simulink model "TRLQR2"  (R2024b)
settings: Solver=VariableStepAuto  StartTime=0.0  StopTime=10.0  RelTol=1e-3
undefined symbols (not defined in the file): start, theta0
settings Model: Creator=mwali  LastModifiedBy=mwali
settings ConfigComp: CovBoundaryAbsTol=1.0e-5

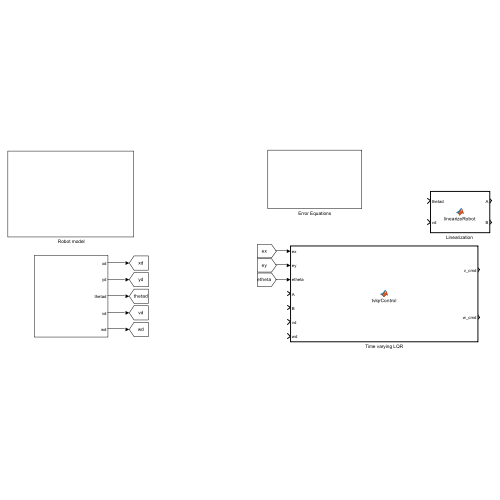
[thumbnail: Simulink's stored preview of the top-level diagram]
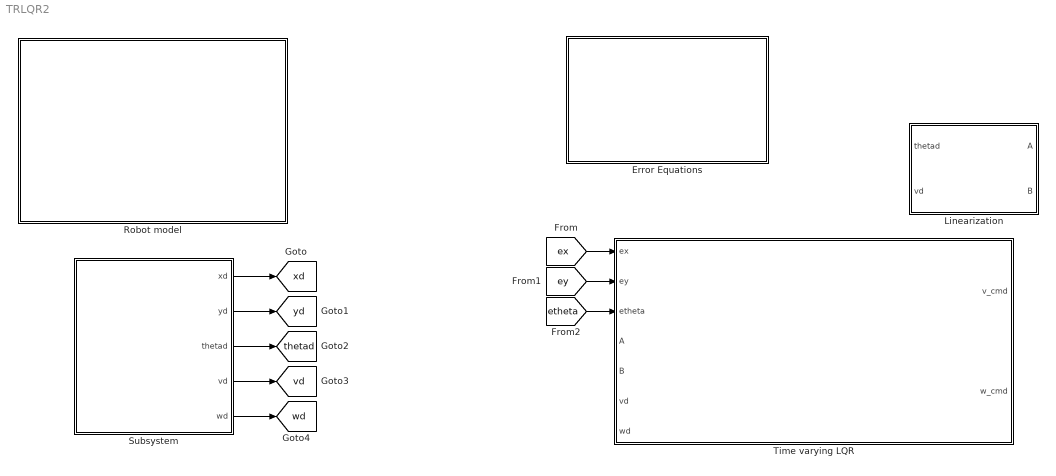
== system TRLQR2 ==
  " Robot model" : Subsystem
  Error Equations : Subsystem
  "Linearization " : MATLAB Function  TreatAsAtomicUnit=on
  Subsystem : Subsystem
  Time varying LQR : MATLAB Function  TreatAsAtomicUnit=on
  tag scope: thetad=global, vd=global, wd=global, xd=global, yd=global
  wires:
  [ex] -> Time varying LQR/1(ex)
  [ey] -> Time varying LQR/2(ey)
  [etheta] -> Time varying LQR/3(etheta)
  Subsystem/1(xd) -> [xd]
  Subsystem/2(yd) -> [yd]
  Subsystem/3(thetad) -> [thetad]
  Subsystem/4(vd) -> [vd]
  Subsystem/5(wd) -> [wd]

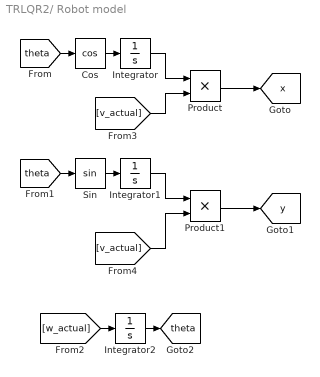
== system TRLQR2/ Robot model ==
  Cos : Trigonometry  Operator=cos
  Integrator : Integrator  InitialCondition=start(1)
  Integrator1 : Integrator  InitialCondition=start(2)
  Integrator2 : Integrator  InitialCondition=theta0
  Product : Product
  Product1 : Product
  Sin : Trigonometry
  tag scope: theta=global, x=global, y=global
  wires:
  Sin/1 -> Integrator1/1
  [theta] -> Sin/1
  Cos/1 -> Integrator/1
  Integrator2/1 -> [theta]
  [theta] -> Cos/1
  [w_actual] -> Integrator2/1
  Integrator/1 -> Product/1
  [v_actual] -> Product/2
  Product/1 -> [x]
  Integrator1/1 -> Product1/1
  [v_actual] -> Product1/2
  Product1/1 -> [y]

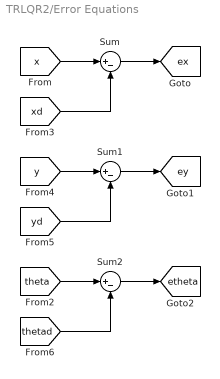
== system TRLQR2/Error Equations ==
  Sum : Sum  Inputs=|+-
  Sum1 : Sum  Inputs=|+-
  Sum2 : Sum  Inputs=|+-
  tag scope: etheta=global, ex=global, ey=global
  wires:
  [y] -> Sum1/1
  Sum/1 -> [ex]
  [x] -> Sum/1
  [yd] -> Sum1/2
  Sum1/1 -> [ey]
  [theta] -> Sum2/1
  [thetad] -> Sum2/2
  Sum2/1 -> [etheta]
  [xd] -> Sum/2

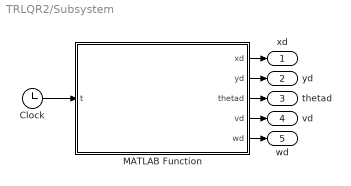
== system TRLQR2/Subsystem ==
  Clock : Clock
  MATLAB Function : MATLAB Function  TreatAsAtomicUnit=on
  xd : Outport
  yd : Outport  Port=2
  thetad : Outport  Port=3
  vd : Outport  Port=4
  wd : Outport  Port=5
  wires:
  Clock/1 -> MATLAB Function/1(t)
  MATLAB Function/4(vd) -> vd/1
  MATLAB Function/1(xd) -> xd/1
  MATLAB Function/5(wd) -> wd/1
  MATLAB Function/2(yd) -> yd/1
  MATLAB Function/3(thetad) -> thetad/1

== matlab function TRLQR2/Linearization  ==
  data: thetad input; A output; vd input; B output
function [A,B] = linearizeRobot(thetad,vd)

A = [0 0 -vd*sin(thetad);
     0 0  vd*cos(thetad);
     0 0  0];

B = [cos(thetad) 0;
     sin(thetad) 0;
     0           1];

== matlab function TRLQR2/Subsystem/MATLAB Function ==
  data: t input; xd output; yd output; thetad output; vd output; wd output
function [xd, yd, thetad, vd, wd] = referenceGenerator(t)

P = evalin('base','P');
theta_ref = evalin('base','theta_ref');
vd_ref = evalin('base','vd_ref');
wd_ref = evalin('base','wd_ref');
Ts_ref = evalin('base','Ts_ref');

idx = floor(t / Ts_ref) + 1;

if idx > size(P,1)
    idx = size(P,1);
end

xd = P(idx,1);
yd = P(idx,2);
thetad = theta_ref(idx);
vd = vd_ref(idx);
wd = wd_ref(idx);

== matlab function TRLQR2/Time varying LQR ==
  data: ex input; v_cmd output; ey input; etheta input; A input; B input; vd input; wd input; w_cmd output
function [v_cmd, w_cmd] = tvlqrControl(ex, ey, etheta, A, B, vd, wd)

Q = diag([10 10 5]);
R = diag([1 1]);

K = lqr(A, B, Q, R);

e = [ex; ey; etheta];
u_corr = -K * e;

v_cmd = vd + u_corr(1);
w_cmd = wd + u_corr(2);
